simulink model "sequentialProcessorNarenKolli"  (R2018b)
settings: Solver=VariableStepAuto  StartTime=0.0  StopTime=10  RelTol=1e-3
libraries: hdlsllib x172, simulink_extras x9
(part 2 of 4)

== system sequentialProcessorNarenKolli/8-Bit_Processor /8-Bit_Subtractor/Full Adder 6  ==
  X : Inport
  Y : Inport  Port=2
  Z : Inport  Port=3
  Half Adder : Subsystem
  Half Adder1 : Subsystem
  OR : Logic  Operator=OR  AllPortsSameDT=off  OutDataTypeStr=boolean
  S : Outport
  C : Outport  Port=2
  wires:
  Half Adder/2(Carry) -> OR/2
  OR/1 -> C/1
  Z/1 -> Half Adder1/2(B)
  X/1 -> Half Adder/1(A)
  Half Adder1/1(Sum) -> S/1
  Half Adder/1(Sum) -> Half Adder1/1(A)
  Y/1 -> Half Adder/2(B)
  Half Adder1/2(Carry) -> OR/1

== system sequentialProcessorNarenKolli/8-Bit_Processor /8-Bit_Subtractor/Full Adder 7  ==
  X : Inport
  Y : Inport  Port=2
  Z : Inport  Port=3
  Half Adder : Subsystem
  Half Adder1 : Subsystem
  OR : Logic  Operator=OR  AllPortsSameDT=off  OutDataTypeStr=boolean
  S : Outport
  C : Outport  Port=2
  wires:
  Half Adder/2(Carry) -> OR/2
  OR/1 -> C/1
  Z/1 -> Half Adder1/2(B)
  X/1 -> Half Adder/1(A)
  Half Adder1/1(Sum) -> S/1
  Half Adder/1(Sum) -> Half Adder1/1(A)
  Y/1 -> Half Adder/2(B)
  Half Adder1/2(Carry) -> OR/1

== system sequentialProcessorNarenKolli/8-Bit_Processor /8-Bit_Subtractor/Slicer 1  ==
  X : Inport  OutDataTypeStr=uint8  SampleTime=1
  Bit Slice : hdlsllib/Logic and Bit Operations/Bit Slice  lidx=7  ridx=7
  Bit Slice1 : hdlsllib/Logic and Bit Operations/Bit Slice  lidx=6  ridx=6
  Bit Slice2 : hdlsllib/Logic and Bit Operations/Bit Slice  lidx=5  ridx=5
  Bit Slice3 : hdlsllib/Logic and Bit Operations/Bit Slice  lidx=4  ridx=4
  Bit Slice4 : hdlsllib/Logic and Bit Operations/Bit Slice  lidx=3  ridx=3
  Bit Slice5 : hdlsllib/Logic and Bit Operations/Bit Slice  lidx=2  ridx=2
  Bit Slice6 : hdlsllib/Logic and Bit Operations/Bit Slice  lidx=1  ridx=1
  Bit Slice7 : hdlsllib/Logic and Bit Operations/Bit Slice  lidx=0  ridx=0
  Data Type Conversion{,1..7} (8 alike) : DataTypeConversion
  Y7 : Outport
  Y6 : Outport  Port=2
  Y5 : Outport  Port=3
  Y4 : Outport  Port=4
  Y3 : Outport  Port=5
  Y2 : Outport  Port=6
  Y1 : Outport  Port=7
  Y0 : Outport  Port=8
  wires:
  Data Type Conversion4/1 -> Y4/1
  Bit Slice3/1 -> Data Type Conversion4/1
  X/1 -> Bit Slice3/1, Bit Slice2/1, Bit Slice1/1, Bit Slice/1, Bit Slice4/1, Bit Slice5/1, Bit Slice6/1, Bit Slice7/1
  Bit Slice1/1 -> Data Type Conversion6/1
  Data Type Conversion1/1 -> Y1/1
  Bit Slice6/1 -> Data Type Conversion1/1
  Bit Slice5/1 -> Data Type Conversion2/1
  Bit Slice2/1 -> Data Type Conversion5/1
  Data Type Conversion/1 -> Y0/1
  Bit Slice4/1 -> Data Type Conversion3/1
  Bit Slice/1 -> Data Type Conversion7/1
  Data Type Conversion7/1 -> Y7/1
  Bit Slice7/1 -> Data Type Conversion/1
  Data Type Conversion3/1 -> Y3/1
  Data Type Conversion5/1 -> Y5/1
  Data Type Conversion6/1 -> Y6/1
  Data Type Conversion2/1 -> Y2/1

== system sequentialProcessorNarenKolli/8-Bit_Processor /8-Bit_Subtractor/Slicer 2  ==
  X : Inport  OutDataTypeStr=uint8  SampleTime=1
  Bit Slice : hdlsllib/Logic and Bit Operations/Bit Slice  lidx=7  ridx=7
  Bit Slice1 : hdlsllib/Logic and Bit Operations/Bit Slice  lidx=6  ridx=6
  Bit Slice2 : hdlsllib/Logic and Bit Operations/Bit Slice  lidx=5  ridx=5
  Bit Slice3 : hdlsllib/Logic and Bit Operations/Bit Slice  lidx=4  ridx=4
  Bit Slice4 : hdlsllib/Logic and Bit Operations/Bit Slice  lidx=3  ridx=3
  Bit Slice5 : hdlsllib/Logic and Bit Operations/Bit Slice  lidx=2  ridx=2
  Bit Slice6 : hdlsllib/Logic and Bit Operations/Bit Slice  lidx=1  ridx=1
  Bit Slice7 : hdlsllib/Logic and Bit Operations/Bit Slice  lidx=0  ridx=0
  Data Type Conversion{,1..7} (8 alike) : DataTypeConversion
  Y7 : Outport
  Y6 : Outport  Port=2
  Y5 : Outport  Port=3
  Y4 : Outport  Port=4
  Y3 : Outport  Port=5
  Y2 : Outport  Port=6
  Y1 : Outport  Port=7
  Y0 : Outport  Port=8
  wires:
  Data Type Conversion4/1 -> Y4/1
  Bit Slice3/1 -> Data Type Conversion4/1
  X/1 -> Bit Slice3/1, Bit Slice2/1, Bit Slice1/1, Bit Slice/1, Bit Slice4/1, Bit Slice5/1, Bit Slice6/1, Bit Slice7/1
  Bit Slice1/1 -> Data Type Conversion6/1
  Data Type Conversion1/1 -> Y1/1
  Bit Slice6/1 -> Data Type Conversion1/1
  Bit Slice5/1 -> Data Type Conversion2/1
  Bit Slice2/1 -> Data Type Conversion5/1
  Data Type Conversion/1 -> Y0/1
  Bit Slice4/1 -> Data Type Conversion3/1
  Bit Slice/1 -> Data Type Conversion7/1
  Data Type Conversion7/1 -> Y7/1
  Bit Slice7/1 -> Data Type Conversion/1
  Data Type Conversion3/1 -> Y3/1
  Data Type Conversion5/1 -> Y5/1
  Data Type Conversion6/1 -> Y6/1
  Data Type Conversion2/1 -> Y2/1

== system sequentialProcessorNarenKolli/8-Bit_Processor /8-bit 4-to-1 MUX/4 x 1 MUX ==
  s : Inport  OutDataTypeStr=int8  SampleTime=1
  "x0 " : Inport  Port=2  OutDataTypeStr=boolean
  x2 : Inport  Port=3  OutDataTypeStr=boolean
  x1 : Inport  Port=4  OutDataTypeStr=boolean
  x3 : Inport  Port=5  OutDataTypeStr=boolean
  AND{,1..3} (4 alike) : Logic  Inputs=3  IconShape=distinctive  AllPortsSameDT=off  OutDataTypeStr=boolean
  Bit Slice : hdlsllib/Logic and Bit Operations/Bit Slice  lidx=1  ridx=1
      settings: SourceProductName=Simulink  SourceProductBaseCode=SL
  Bit Slice1 : hdlsllib/Logic and Bit Operations/Bit Slice  lidx=0  ridx=0
      settings: SourceProductName=Simulink  SourceProductBaseCode=SL
  Data Type Conversion : DataTypeConversion  OutDataTypeStr=boolean
  Data Type Conversion1 : DataTypeConversion  OutDataTypeStr=boolean
  NOT S0 : Logic  Operator=NOT  IconShape=distinctive  AllPortsSameDT=off  OutDataTypeStr=boolean
  NOT S1 : Logic  Operator=NOT  IconShape=distinctive  AllPortsSameDT=off  OutDataTypeStr=boolean
  OR : Logic  Operator=OR  Inputs=4  IconShape=distinctive  AllPortsSameDT=off  OutDataTypeStr=boolean
  y : Outport  VectorParamsAs1DForOutWhenUnconnected=on
  wires:
  Data Type Conversion/1 -> AND3/1, AND2/1, NOT S1/1
  Data Type Conversion1/1 -> AND3/2, AND1/2, NOT S0/1
  NOT S0/1 -> AND2/2, AND/2
  x1/1 -> AND1/3
  x2/1 -> AND2/3
  AND3/1 -> OR/4
  NOT S1/1 -> AND1/1, AND/1
  x3/1 -> AND3/3
  AND2/1 -> OR/3
  AND1/1 -> OR/2
  "x0 "/1 -> AND/3
  Bit Slice1/1 -> Data Type Conversion1/1
  s/1 -> Bit Slice/1, Bit Slice1/1
  Bit Slice/1 -> Data Type Conversion/1
  AND/1 -> OR/1
  OR/1 -> y/1

== system sequentialProcessorNarenKolli/8-Bit_Processor /8-bit 4-to-1 MUX/4 x 1 MUX1 ==
  s : Inport  OutDataTypeStr=int8  SampleTime=1
  "x0 " : Inport  Port=2  OutDataTypeStr=boolean
  x2 : Inport  Port=3  OutDataTypeStr=boolean
  x1 : Inport  Port=4  OutDataTypeStr=boolean
  x3 : Inport  Port=5  OutDataTypeStr=boolean
  AND{,1..3} (4 alike) : Logic  Inputs=3  IconShape=distinctive  AllPortsSameDT=off  OutDataTypeStr=boolean
  Bit Slice : hdlsllib/Logic and Bit Operations/Bit Slice  lidx=1  ridx=1
      settings: SourceProductName=Simulink  SourceProductBaseCode=SL
  Bit Slice1 : hdlsllib/Logic and Bit Operations/Bit Slice  lidx=0  ridx=0
      settings: SourceProductName=Simulink  SourceProductBaseCode=SL
  Data Type Conversion : DataTypeConversion  OutDataTypeStr=boolean
  Data Type Conversion1 : DataTypeConversion  OutDataTypeStr=boolean
  NOT S0 : Logic  Operator=NOT  IconShape=distinctive  AllPortsSameDT=off  OutDataTypeStr=boolean
  NOT S1 : Logic  Operator=NOT  IconShape=distinctive  AllPortsSameDT=off  OutDataTypeStr=boolean
  OR : Logic  Operator=OR  Inputs=4  IconShape=distinctive  AllPortsSameDT=off  OutDataTypeStr=boolean
  y : Outport  VectorParamsAs1DForOutWhenUnconnected=on
  wires:
  Data Type Conversion/1 -> AND3/1, AND2/1, NOT S1/1
  Data Type Conversion1/1 -> AND3/2, AND1/2, NOT S0/1
  NOT S0/1 -> AND2/2, AND/2
  x1/1 -> AND1/3
  x2/1 -> AND2/3
  AND3/1 -> OR/4
  NOT S1/1 -> AND1/1, AND/1
  x3/1 -> AND3/3
  AND2/1 -> OR/3
  AND1/1 -> OR/2
  "x0 "/1 -> AND/3
  Bit Slice1/1 -> Data Type Conversion1/1
  s/1 -> Bit Slice/1, Bit Slice1/1
  Bit Slice/1 -> Data Type Conversion/1
  AND/1 -> OR/1
  OR/1 -> y/1

== system sequentialProcessorNarenKolli/8-Bit_Processor /8-bit 4-to-1 MUX/4 x 1 MUX2 ==
  s : Inport  OutDataTypeStr=int8  SampleTime=1
  "x0 " : Inport  Port=2  OutDataTypeStr=boolean
  x2 : Inport  Port=3  OutDataTypeStr=boolean
  x1 : Inport  Port=4  OutDataTypeStr=boolean
  x3 : Inport  Port=5  OutDataTypeStr=boolean
  AND{,1..3} (4 alike) : Logic  Inputs=3  IconShape=distinctive  AllPortsSameDT=off  OutDataTypeStr=boolean
  Bit Slice : hdlsllib/Logic and Bit Operations/Bit Slice  lidx=1  ridx=1
      settings: SourceProductName=Simulink  SourceProductBaseCode=SL
  Bit Slice1 : hdlsllib/Logic and Bit Operations/Bit Slice  lidx=0  ridx=0
      settings: SourceProductName=Simulink  SourceProductBaseCode=SL
  Data Type Conversion : DataTypeConversion  OutDataTypeStr=boolean
  Data Type Conversion1 : DataTypeConversion  OutDataTypeStr=boolean
  NOT S0 : Logic  Operator=NOT  IconShape=distinctive  AllPortsSameDT=off  OutDataTypeStr=boolean
  NOT S1 : Logic  Operator=NOT  IconShape=distinctive  AllPortsSameDT=off  OutDataTypeStr=boolean
  OR : Logic  Operator=OR  Inputs=4  IconShape=distinctive  AllPortsSameDT=off  OutDataTypeStr=boolean
  y : Outport  VectorParamsAs1DForOutWhenUnconnected=on
  wires:
  Data Type Conversion/1 -> AND3/1, AND2/1, NOT S1/1
  Data Type Conversion1/1 -> AND3/2, AND1/2, NOT S0/1
  NOT S0/1 -> AND2/2, AND/2
  x1/1 -> AND1/3
  x2/1 -> AND2/3
  AND3/1 -> OR/4
  NOT S1/1 -> AND1/1, AND/1
  x3/1 -> AND3/3
  AND2/1 -> OR/3
  AND1/1 -> OR/2
  "x0 "/1 -> AND/3
  Bit Slice1/1 -> Data Type Conversion1/1
  s/1 -> Bit Slice/1, Bit Slice1/1
  Bit Slice/1 -> Data Type Conversion/1
  AND/1 -> OR/1
  OR/1 -> y/1

== system sequentialProcessorNarenKolli/8-Bit_Processor /8-bit 4-to-1 MUX/4 x 1 MUX3 ==
  s : Inport  OutDataTypeStr=int8  SampleTime=1
  "x0 " : Inport  Port=2  OutDataTypeStr=boolean
  x2 : Inport  Port=3  OutDataTypeStr=boolean
  x1 : Inport  Port=4  OutDataTypeStr=boolean
  x3 : Inport  Port=5  OutDataTypeStr=boolean
  AND{,1..3} (4 alike) : Logic  Inputs=3  IconShape=distinctive  AllPortsSameDT=off  OutDataTypeStr=boolean
  Bit Slice : hdlsllib/Logic and Bit Operations/Bit Slice  lidx=1  ridx=1
      settings: SourceProductName=Simulink  SourceProductBaseCode=SL
  Bit Slice1 : hdlsllib/Logic and Bit Operations/Bit Slice  lidx=0  ridx=0
      settings: SourceProductName=Simulink  SourceProductBaseCode=SL
  Data Type Conversion : DataTypeConversion  OutDataTypeStr=boolean
  Data Type Conversion1 : DataTypeConversion  OutDataTypeStr=boolean
  NOT S0 : Logic  Operator=NOT  IconShape=distinctive  AllPortsSameDT=off  OutDataTypeStr=boolean
  NOT S1 : Logic  Operator=NOT  IconShape=distinctive  AllPortsSameDT=off  OutDataTypeStr=boolean
  OR : Logic  Operator=OR  Inputs=4  IconShape=distinctive  AllPortsSameDT=off  OutDataTypeStr=boolean
  y : Outport  VectorParamsAs1DForOutWhenUnconnected=on
  wires:
  Data Type Conversion/1 -> AND3/1, AND2/1, NOT S1/1
  Data Type Conversion1/1 -> AND3/2, AND1/2, NOT S0/1
  NOT S0/1 -> AND2/2, AND/2
  x1/1 -> AND1/3
  x2/1 -> AND2/3
  AND3/1 -> OR/4
  NOT S1/1 -> AND1/1, AND/1
  x3/1 -> AND3/3
  AND2/1 -> OR/3
  AND1/1 -> OR/2
  "x0 "/1 -> AND/3
  Bit Slice1/1 -> Data Type Conversion1/1
  s/1 -> Bit Slice/1, Bit Slice1/1
  Bit Slice/1 -> Data Type Conversion/1
  AND/1 -> OR/1
  OR/1 -> y/1

== system sequentialProcessorNarenKolli/8-Bit_Processor /8-bit 4-to-1 MUX/4 x 1 MUX4 ==
  s : Inport  OutDataTypeStr=int8  SampleTime=1
  "x0 " : Inport  Port=2  OutDataTypeStr=boolean
  x2 : Inport  Port=3  OutDataTypeStr=boolean
  x1 : Inport  Port=4  OutDataTypeStr=boolean
  x3 : Inport  Port=5  OutDataTypeStr=boolean
  AND{,1..3} (4 alike) : Logic  Inputs=3  IconShape=distinctive  AllPortsSameDT=off  OutDataTypeStr=boolean
  Bit Slice : hdlsllib/Logic and Bit Operations/Bit Slice  lidx=1  ridx=1
      settings: SourceProductName=Simulink  SourceProductBaseCode=SL
  Bit Slice1 : hdlsllib/Logic and Bit Operations/Bit Slice  lidx=0  ridx=0
      settings: SourceProductName=Simulink  SourceProductBaseCode=SL
  Data Type Conversion : DataTypeConversion  OutDataTypeStr=boolean
  Data Type Conversion1 : DataTypeConversion  OutDataTypeStr=boolean
  NOT S0 : Logic  Operator=NOT  IconShape=distinctive  AllPortsSameDT=off  OutDataTypeStr=boolean
  NOT S1 : Logic  Operator=NOT  IconShape=distinctive  AllPortsSameDT=off  OutDataTypeStr=boolean
  OR : Logic  Operator=OR  Inputs=4  IconShape=distinctive  AllPortsSameDT=off  OutDataTypeStr=boolean
  y : Outport  VectorParamsAs1DForOutWhenUnconnected=on
  wires:
  Data Type Conversion/1 -> AND3/1, AND2/1, NOT S1/1
  Data Type Conversion1/1 -> AND3/2, AND1/2, NOT S0/1
  NOT S0/1 -> AND2/2, AND/2
  x1/1 -> AND1/3
  x2/1 -> AND2/3
  AND3/1 -> OR/4
  NOT S1/1 -> AND1/1, AND/1
  x3/1 -> AND3/3
  AND2/1 -> OR/3
  AND1/1 -> OR/2
  "x0 "/1 -> AND/3
  Bit Slice1/1 -> Data Type Conversion1/1
  s/1 -> Bit Slice/1, Bit Slice1/1
  Bit Slice/1 -> Data Type Conversion/1
  AND/1 -> OR/1
  OR/1 -> y/1

== system sequentialProcessorNarenKolli/8-Bit_Processor /8-bit 4-to-1 MUX/4 x 1 MUX5 ==
  s : Inport  OutDataTypeStr=int8  SampleTime=1
  "x0 " : Inport  Port=2  OutDataTypeStr=boolean
  x2 : Inport  Port=3  OutDataTypeStr=boolean
  x1 : Inport  Port=4  OutDataTypeStr=boolean
  x3 : Inport  Port=5  OutDataTypeStr=boolean
  AND{,1..3} (4 alike) : Logic  Inputs=3  IconShape=distinctive  AllPortsSameDT=off  OutDataTypeStr=boolean
  Bit Slice : hdlsllib/Logic and Bit Operations/Bit Slice  lidx=1  ridx=1
      settings: SourceProductName=Simulink  SourceProductBaseCode=SL
  Bit Slice1 : hdlsllib/Logic and Bit Operations/Bit Slice  lidx=0  ridx=0
      settings: SourceProductName=Simulink  SourceProductBaseCode=SL
  Data Type Conversion : DataTypeConversion  OutDataTypeStr=boolean
  Data Type Conversion1 : DataTypeConversion  OutDataTypeStr=boolean
  NOT S0 : Logic  Operator=NOT  IconShape=distinctive  AllPortsSameDT=off  OutDataTypeStr=boolean
  NOT S1 : Logic  Operator=NOT  IconShape=distinctive  AllPortsSameDT=off  OutDataTypeStr=boolean
  OR : Logic  Operator=OR  Inputs=4  IconShape=distinctive  AllPortsSameDT=off  OutDataTypeStr=boolean
  y : Outport  VectorParamsAs1DForOutWhenUnconnected=on
  wires:
  Data Type Conversion/1 -> AND3/1, AND2/1, NOT S1/1
  Data Type Conversion1/1 -> AND3/2, AND1/2, NOT S0/1
  NOT S0/1 -> AND2/2, AND/2
  x1/1 -> AND1/3
  x2/1 -> AND2/3
  AND3/1 -> OR/4
  NOT S1/1 -> AND1/1, AND/1
  x3/1 -> AND3/3
  AND2/1 -> OR/3
  AND1/1 -> OR/2
  "x0 "/1 -> AND/3
  Bit Slice1/1 -> Data Type Conversion1/1
  s/1 -> Bit Slice/1, Bit Slice1/1
  Bit Slice/1 -> Data Type Conversion/1
  AND/1 -> OR/1
  OR/1 -> y/1

== system sequentialProcessorNarenKolli/8-Bit_Processor /8-bit 4-to-1 MUX/4 x 1 MUX6 ==
  s : Inport  OutDataTypeStr=int8  SampleTime=1
  "x0 " : Inport  Port=2  OutDataTypeStr=boolean
  x2 : Inport  Port=3  OutDataTypeStr=boolean
  x1 : Inport  Port=4  OutDataTypeStr=boolean
  x3 : Inport  Port=5  OutDataTypeStr=boolean
  AND{,1..3} (4 alike) : Logic  Inputs=3  IconShape=distinctive  AllPortsSameDT=off  OutDataTypeStr=boolean
  Bit Slice : hdlsllib/Logic and Bit Operations/Bit Slice  lidx=1  ridx=1
      settings: SourceProductName=Simulink  SourceProductBaseCode=SL
  Bit Slice1 : hdlsllib/Logic and Bit Operations/Bit Slice  lidx=0  ridx=0
      settings: SourceProductName=Simulink  SourceProductBaseCode=SL
  Data Type Conversion : DataTypeConversion  OutDataTypeStr=boolean
  Data Type Conversion1 : DataTypeConversion  OutDataTypeStr=boolean
  NOT S0 : Logic  Operator=NOT  IconShape=distinctive  AllPortsSameDT=off  OutDataTypeStr=boolean
  NOT S1 : Logic  Operator=NOT  IconShape=distinctive  AllPortsSameDT=off  OutDataTypeStr=boolean
  OR : Logic  Operator=OR  Inputs=4  IconShape=distinctive  AllPortsSameDT=off  OutDataTypeStr=boolean
  y : Outport  VectorParamsAs1DForOutWhenUnconnected=on
  wires:
  Data Type Conversion/1 -> AND3/1, AND2/1, NOT S1/1
  Data Type Conversion1/1 -> AND3/2, AND1/2, NOT S0/1
  NOT S0/1 -> AND2/2, AND/2
  x1/1 -> AND1/3
  x2/1 -> AND2/3
  AND3/1 -> OR/4
  NOT S1/1 -> AND1/1, AND/1
  x3/1 -> AND3/3
  AND2/1 -> OR/3
  AND1/1 -> OR/2
  "x0 "/1 -> AND/3
  Bit Slice1/1 -> Data Type Conversion1/1
  s/1 -> Bit Slice/1, Bit Slice1/1
  Bit Slice/1 -> Data Type Conversion/1
  AND/1 -> OR/1
  OR/1 -> y/1

== system sequentialProcessorNarenKolli/8-Bit_Processor /8-bit 4-to-1 MUX/4 x 1 MUX7 ==
  s : Inport  OutDataTypeStr=int8  SampleTime=1
  "x0 " : Inport  Port=2  OutDataTypeStr=boolean
  x2 : Inport  Port=3  OutDataTypeStr=boolean
  x1 : Inport  Port=4  OutDataTypeStr=boolean
  x3 : Inport  Port=5  OutDataTypeStr=boolean
  AND{,1..3} (4 alike) : Logic  Inputs=3  IconShape=distinctive  AllPortsSameDT=off  OutDataTypeStr=boolean
  Bit Slice : hdlsllib/Logic and Bit Operations/Bit Slice  lidx=1  ridx=1
      settings: SourceProductName=Simulink  SourceProductBaseCode=SL
  Bit Slice1 : hdlsllib/Logic and Bit Operations/Bit Slice  lidx=0  ridx=0
      settings: SourceProductName=Simulink  SourceProductBaseCode=SL
  Data Type Conversion : DataTypeConversion  OutDataTypeStr=boolean
  Data Type Conversion1 : DataTypeConversion  OutDataTypeStr=boolean
  NOT S0 : Logic  Operator=NOT  IconShape=distinctive  AllPortsSameDT=off  OutDataTypeStr=boolean
  NOT S1 : Logic  Operator=NOT  IconShape=distinctive  AllPortsSameDT=off  OutDataTypeStr=boolean
  OR : Logic  Operator=OR  Inputs=4  IconShape=distinctive  AllPortsSameDT=off  OutDataTypeStr=boolean
  y : Outport  VectorParamsAs1DForOutWhenUnconnected=on
  wires:
  Data Type Conversion/1 -> AND3/1, AND2/1, NOT S1/1
  Data Type Conversion1/1 -> AND3/2, AND1/2, NOT S0/1
  NOT S0/1 -> AND2/2, AND/2
  x1/1 -> AND1/3
  x2/1 -> AND2/3
  AND3/1 -> OR/4
  NOT S1/1 -> AND1/1, AND/1
  x3/1 -> AND3/3
  AND2/1 -> OR/3
  AND1/1 -> OR/2
  "x0 "/1 -> AND/3
  Bit Slice1/1 -> Data Type Conversion1/1
  s/1 -> Bit Slice/1, Bit Slice1/1
  Bit Slice/1 -> Data Type Conversion/1
  AND/1 -> OR/1
  OR/1 -> y/1

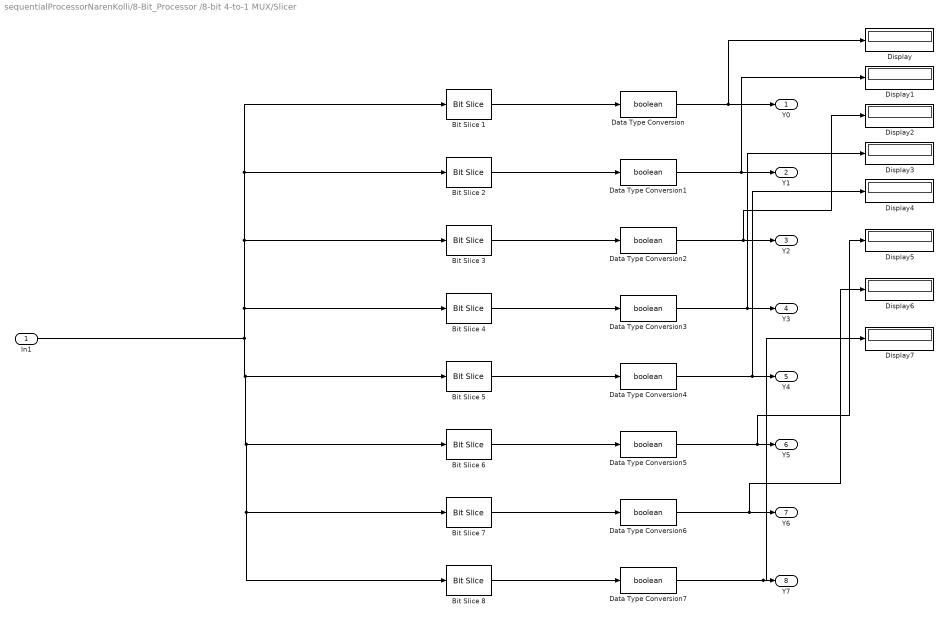
== system sequentialProcessorNarenKolli/8-Bit_Processor /8-bit 4-to-1 MUX/Slicer ==
  In1 : Inport
  Bit Slice 1 : hdlsllib/Logic and Bit Operations/Bit Slice  lidx=0  ridx=0
      settings: SourceProductName=Simulink  SourceProductBaseCode=SL
  "Bit Slice 2 " : hdlsllib/Logic and Bit Operations/Bit Slice  lidx=1  ridx=1
      settings: SourceProductName=Simulink  SourceProductBaseCode=SL
  Bit Slice 3 : hdlsllib/Logic and Bit Operations/Bit Slice  lidx=2  ridx=2
      settings: SourceProductName=Simulink  SourceProductBaseCode=SL
  Bit Slice 4 : hdlsllib/Logic and Bit Operations/Bit Slice  lidx=3  ridx=3
      settings: SourceProductName=Simulink  SourceProductBaseCode=SL
  Bit Slice 5 : hdlsllib/Logic and Bit Operations/Bit Slice  lidx=4  ridx=4
      settings: SourceProductName=Simulink  SourceProductBaseCode=SL
  Bit Slice 6 : hdlsllib/Logic and Bit Operations/Bit Slice  lidx=5  ridx=5
      settings: SourceProductName=Simulink  SourceProductBaseCode=SL
  Bit Slice 7 : hdlsllib/Logic and Bit Operations/Bit Slice  lidx=6  ridx=6
      settings: SourceProductName=Simulink  SourceProductBaseCode=SL
  Bit Slice 8 : hdlsllib/Logic and Bit Operations/Bit Slice  lidx=7  ridx=7
      settings: SourceProductName=Simulink  SourceProductBaseCode=SL
  Data Type Conversion{,1..7} (8 alike) : DataTypeConversion  OutDataTypeStr=boolean
  Display{,1..7} (8 alike) : Display
  Y0 : Outport  VectorParamsAs1DForOutWhenUnconnected=on
  Y1 : Outport  Port=2  VectorParamsAs1DForOutWhenUnconnected=on
  Y2 : Outport  Port=3  VectorParamsAs1DForOutWhenUnconnected=on
  Y3 : Outport  Port=4  VectorParamsAs1DForOutWhenUnconnected=on
  Y4 : Outport  Port=5  VectorParamsAs1DForOutWhenUnconnected=on
  Y5 : Outport  Port=6  VectorParamsAs1DForOutWhenUnconnected=on
  Y6 : Outport  Port=7  VectorParamsAs1DForOutWhenUnconnected=on
  Y7 : Outport  Port=8  VectorParamsAs1DForOutWhenUnconnected=on
  wires:
  Data Type Conversion2/1 -> Display2/1, Y2/1
  Data Type Conversion/1 -> Display/1, Y0/1
  Bit Slice 4/1 -> Data Type Conversion3/1
  Data Type Conversion7/1 -> Display7/1, Y7/1
  Bit Slice 3/1 -> Data Type Conversion2/1
  Bit Slice 8/1 -> Data Type Conversion7/1
  Bit Slice 1/1 -> Data Type Conversion/1
  Bit Slice 6/1 -> Data Type Conversion5/1
  Data Type Conversion1/1 -> Display1/1, Y1/1
  "Bit Slice 2 "/1 -> Data Type Conversion1/1
  Data Type Conversion3/1 -> Display3/1, Y3/1
  Data Type Conversion5/1 -> Display5/1, Y5/1
  Data Type Conversion6/1 -> Display6/1, Y6/1
  Data Type Conversion4/1 -> Display4/1, Y4/1
  Bit Slice 5/1 -> Data Type Conversion4/1
  Bit Slice 7/1 -> Data Type Conversion6/1
  In1/1 -> Bit Slice 4/1, Bit Slice 3/1, "Bit Slice 2 "/1, Bit Slice 1/1, Bit Slice 8/1, Bit Slice 7/1, Bit Slice 6/1, Bit Slice 5/1

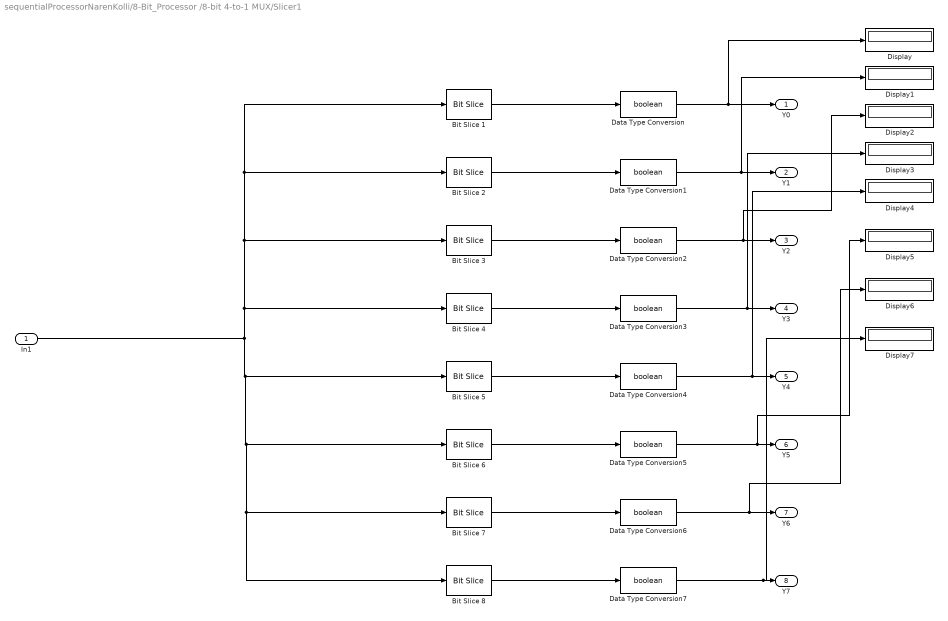
== system sequentialProcessorNarenKolli/8-Bit_Processor /8-bit 4-to-1 MUX/Slicer1 ==
  In1 : Inport
  Bit Slice 1 : hdlsllib/Logic and Bit Operations/Bit Slice  lidx=0  ridx=0
      settings: SourceProductName=Simulink  SourceProductBaseCode=SL
  "Bit Slice 2 " : hdlsllib/Logic and Bit Operations/Bit Slice  lidx=1  ridx=1
      settings: SourceProductName=Simulink  SourceProductBaseCode=SL
  Bit Slice 3 : hdlsllib/Logic and Bit Operations/Bit Slice  lidx=2  ridx=2
      settings: SourceProductName=Simulink  SourceProductBaseCode=SL
  Bit Slice 4 : hdlsllib/Logic and Bit Operations/Bit Slice  lidx=3  ridx=3
      settings: SourceProductName=Simulink  SourceProductBaseCode=SL
  Bit Slice 5 : hdlsllib/Logic and Bit Operations/Bit Slice  lidx=4  ridx=4
      settings: SourceProductName=Simulink  SourceProductBaseCode=SL
  Bit Slice 6 : hdlsllib/Logic and Bit Operations/Bit Slice  lidx=5  ridx=5
      settings: SourceProductName=Simulink  SourceProductBaseCode=SL
  Bit Slice 7 : hdlsllib/Logic and Bit Operations/Bit Slice  lidx=6  ridx=6
      settings: SourceProductName=Simulink  SourceProductBaseCode=SL
  Bit Slice 8 : hdlsllib/Logic and Bit Operations/Bit Slice  lidx=7  ridx=7
      settings: SourceProductName=Simulink  SourceProductBaseCode=SL
  Data Type Conversion{,1..7} (8 alike) : DataTypeConversion  OutDataTypeStr=boolean
  Display{,1..7} (8 alike) : Display
  Y0 : Outport  VectorParamsAs1DForOutWhenUnconnected=on
  Y1 : Outport  Port=2  VectorParamsAs1DForOutWhenUnconnected=on
  Y2 : Outport  Port=3  VectorParamsAs1DForOutWhenUnconnected=on
  Y3 : Outport  Port=4  VectorParamsAs1DForOutWhenUnconnected=on
  Y4 : Outport  Port=5  VectorParamsAs1DForOutWhenUnconnected=on
  Y5 : Outport  Port=6  VectorParamsAs1DForOutWhenUnconnected=on
  Y6 : Outport  Port=7  VectorParamsAs1DForOutWhenUnconnected=on
  Y7 : Outport  Port=8  VectorParamsAs1DForOutWhenUnconnected=on
  wires:
  Data Type Conversion2/1 -> Display2/1, Y2/1
  Data Type Conversion/1 -> Display/1, Y0/1
  Bit Slice 4/1 -> Data Type Conversion3/1
  Data Type Conversion7/1 -> Display7/1, Y7/1
  Bit Slice 3/1 -> Data Type Conversion2/1
  Bit Slice 8/1 -> Data Type Conversion7/1
  Bit Slice 1/1 -> Data Type Conversion/1
  Bit Slice 6/1 -> Data Type Conversion5/1
  Data Type Conversion1/1 -> Display1/1, Y1/1
  "Bit Slice 2 "/1 -> Data Type Conversion1/1
  Data Type Conversion3/1 -> Display3/1, Y3/1
  Data Type Conversion5/1 -> Display5/1, Y5/1
  Data Type Conversion6/1 -> Display6/1, Y6/1
  Data Type Conversion4/1 -> Display4/1, Y4/1
  Bit Slice 5/1 -> Data Type Conversion4/1
  Bit Slice 7/1 -> Data Type Conversion6/1
  In1/1 -> Bit Slice 4/1, Bit Slice 3/1, "Bit Slice 2 "/1, Bit Slice 1/1, Bit Slice 8/1, Bit Slice 7/1, Bit Slice 6/1, Bit Slice 5/1

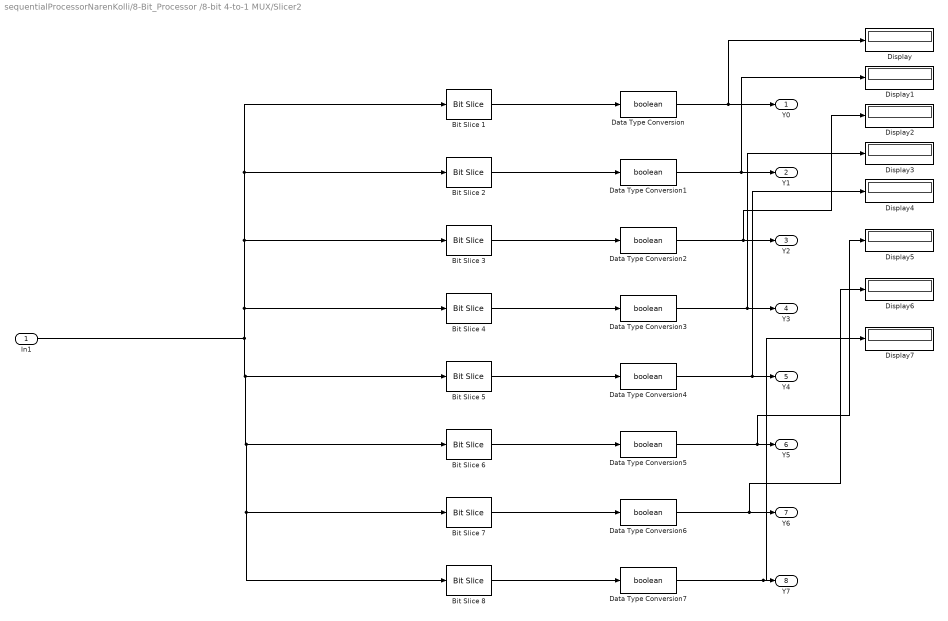
== system sequentialProcessorNarenKolli/8-Bit_Processor /8-bit 4-to-1 MUX/Slicer2 ==
  In1 : Inport
  Bit Slice 1 : hdlsllib/Logic and Bit Operations/Bit Slice  lidx=0  ridx=0
      settings: SourceProductName=Simulink  SourceProductBaseCode=SL
  "Bit Slice 2 " : hdlsllib/Logic and Bit Operations/Bit Slice  lidx=1  ridx=1
      settings: SourceProductName=Simulink  SourceProductBaseCode=SL
  Bit Slice 3 : hdlsllib/Logic and Bit Operations/Bit Slice  lidx=2  ridx=2
      settings: SourceProductName=Simulink  SourceProductBaseCode=SL
  Bit Slice 4 : hdlsllib/Logic and Bit Operations/Bit Slice  lidx=3  ridx=3
      settings: SourceProductName=Simulink  SourceProductBaseCode=SL
  Bit Slice 5 : hdlsllib/Logic and Bit Operations/Bit Slice  lidx=4  ridx=4
      settings: SourceProductName=Simulink  SourceProductBaseCode=SL
  Bit Slice 6 : hdlsllib/Logic and Bit Operations/Bit Slice  lidx=5  ridx=5
      settings: SourceProductName=Simulink  SourceProductBaseCode=SL
  Bit Slice 7 : hdlsllib/Logic and Bit Operations/Bit Slice  lidx=6  ridx=6
      settings: SourceProductName=Simulink  SourceProductBaseCode=SL
  Bit Slice 8 : hdlsllib/Logic and Bit Operations/Bit Slice  lidx=7  ridx=7
      settings: SourceProductName=Simulink  SourceProductBaseCode=SL
  Data Type Conversion{,1..7} (8 alike) : DataTypeConversion  OutDataTypeStr=boolean
  Display{,1..7} (8 alike) : Display
  Y0 : Outport  VectorParamsAs1DForOutWhenUnconnected=on
  Y1 : Outport  Port=2  VectorParamsAs1DForOutWhenUnconnected=on
  Y2 : Outport  Port=3  VectorParamsAs1DForOutWhenUnconnected=on
  Y3 : Outport  Port=4  VectorParamsAs1DForOutWhenUnconnected=on
  Y4 : Outport  Port=5  VectorParamsAs1DForOutWhenUnconnected=on
  Y5 : Outport  Port=6  VectorParamsAs1DForOutWhenUnconnected=on
  Y6 : Outport  Port=7  VectorParamsAs1DForOutWhenUnconnected=on
  Y7 : Outport  Port=8  VectorParamsAs1DForOutWhenUnconnected=on
  wires:
  Data Type Conversion2/1 -> Display2/1, Y2/1
  Data Type Conversion/1 -> Display/1, Y0/1
  Bit Slice 4/1 -> Data Type Conversion3/1
  Data Type Conversion7/1 -> Display7/1, Y7/1
  Bit Slice 3/1 -> Data Type Conversion2/1
  Bit Slice 8/1 -> Data Type Conversion7/1
  Bit Slice 1/1 -> Data Type Conversion/1
  Bit Slice 6/1 -> Data Type Conversion5/1
  Data Type Conversion1/1 -> Display1/1, Y1/1
  "Bit Slice 2 "/1 -> Data Type Conversion1/1
  Data Type Conversion3/1 -> Display3/1, Y3/1
  Data Type Conversion5/1 -> Display5/1, Y5/1
  Data Type Conversion6/1 -> Display6/1, Y6/1
  Data Type Conversion4/1 -> Display4/1, Y4/1
  Bit Slice 5/1 -> Data Type Conversion4/1
  Bit Slice 7/1 -> Data Type Conversion6/1
  In1/1 -> Bit Slice 4/1, Bit Slice 3/1, "Bit Slice 2 "/1, Bit Slice 1/1, Bit Slice 8/1, Bit Slice 7/1, Bit Slice 6/1, Bit Slice 5/1

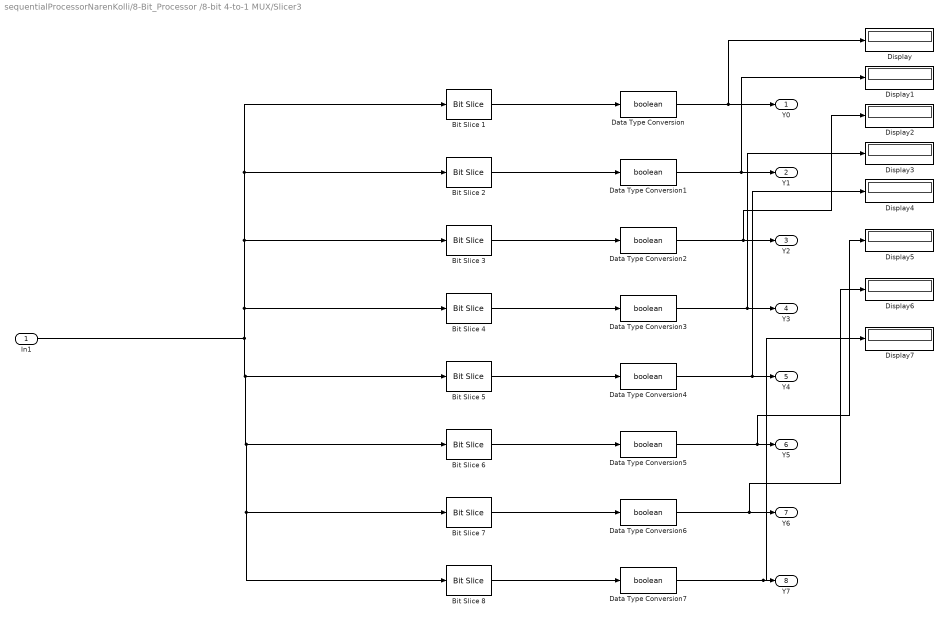
== system sequentialProcessorNarenKolli/8-Bit_Processor /8-bit 4-to-1 MUX/Slicer3 ==
  In1 : Inport
  Bit Slice 1 : hdlsllib/Logic and Bit Operations/Bit Slice  lidx=0  ridx=0
      settings: SourceProductName=Simulink  SourceProductBaseCode=SL
  "Bit Slice 2 " : hdlsllib/Logic and Bit Operations/Bit Slice  lidx=1  ridx=1
      settings: SourceProductName=Simulink  SourceProductBaseCode=SL
  Bit Slice 3 : hdlsllib/Logic and Bit Operations/Bit Slice  lidx=2  ridx=2
      settings: SourceProductName=Simulink  SourceProductBaseCode=SL
  Bit Slice 4 : hdlsllib/Logic and Bit Operations/Bit Slice  lidx=3  ridx=3
      settings: SourceProductName=Simulink  SourceProductBaseCode=SL
  Bit Slice 5 : hdlsllib/Logic and Bit Operations/Bit Slice  lidx=4  ridx=4
      settings: SourceProductName=Simulink  SourceProductBaseCode=SL
  Bit Slice 6 : hdlsllib/Logic and Bit Operations/Bit Slice  lidx=5  ridx=5
      settings: SourceProductName=Simulink  SourceProductBaseCode=SL
  Bit Slice 7 : hdlsllib/Logic and Bit Operations/Bit Slice  lidx=6  ridx=6
      settings: SourceProductName=Simulink  SourceProductBaseCode=SL
  Bit Slice 8 : hdlsllib/Logic and Bit Operations/Bit Slice  lidx=7  ridx=7
      settings: SourceProductName=Simulink  SourceProductBaseCode=SL
  Data Type Conversion{,1..7} (8 alike) : DataTypeConversion  OutDataTypeStr=boolean
  Display{,1..7} (8 alike) : Display
  Y0 : Outport  VectorParamsAs1DForOutWhenUnconnected=on
  Y1 : Outport  Port=2  VectorParamsAs1DForOutWhenUnconnected=on
  Y2 : Outport  Port=3  VectorParamsAs1DForOutWhenUnconnected=on
  Y3 : Outport  Port=4  VectorParamsAs1DForOutWhenUnconnected=on
  Y4 : Outport  Port=5  VectorParamsAs1DForOutWhenUnconnected=on
  Y5 : Outport  Port=6  VectorParamsAs1DForOutWhenUnconnected=on
  Y6 : Outport  Port=7  VectorParamsAs1DForOutWhenUnconnected=on
  Y7 : Outport  Port=8  VectorParamsAs1DForOutWhenUnconnected=on
  wires:
  Data Type Conversion2/1 -> Display2/1, Y2/1
  Data Type Conversion/1 -> Display/1, Y0/1
  Bit Slice 4/1 -> Data Type Conversion3/1
  Data Type Conversion7/1 -> Display7/1, Y7/1
  Bit Slice 3/1 -> Data Type Conversion2/1
  Bit Slice 8/1 -> Data Type Conversion7/1
  Bit Slice 1/1 -> Data Type Conversion/1
  Bit Slice 6/1 -> Data Type Conversion5/1
  Data Type Conversion1/1 -> Display1/1, Y1/1
  "Bit Slice 2 "/1 -> Data Type Conversion1/1
  Data Type Conversion3/1 -> Display3/1, Y3/1
  Data Type Conversion5/1 -> Display5/1, Y5/1
  Data Type Conversion6/1 -> Display6/1, Y6/1
  Data Type Conversion4/1 -> Display4/1, Y4/1
  Bit Slice 5/1 -> Data Type Conversion4/1
  Bit Slice 7/1 -> Data Type Conversion6/1
  In1/1 -> Bit Slice 4/1, Bit Slice 3/1, "Bit Slice 2 "/1, Bit Slice 1/1, Bit Slice 8/1, Bit Slice 7/1, Bit Slice 6/1, Bit Slice 5/1

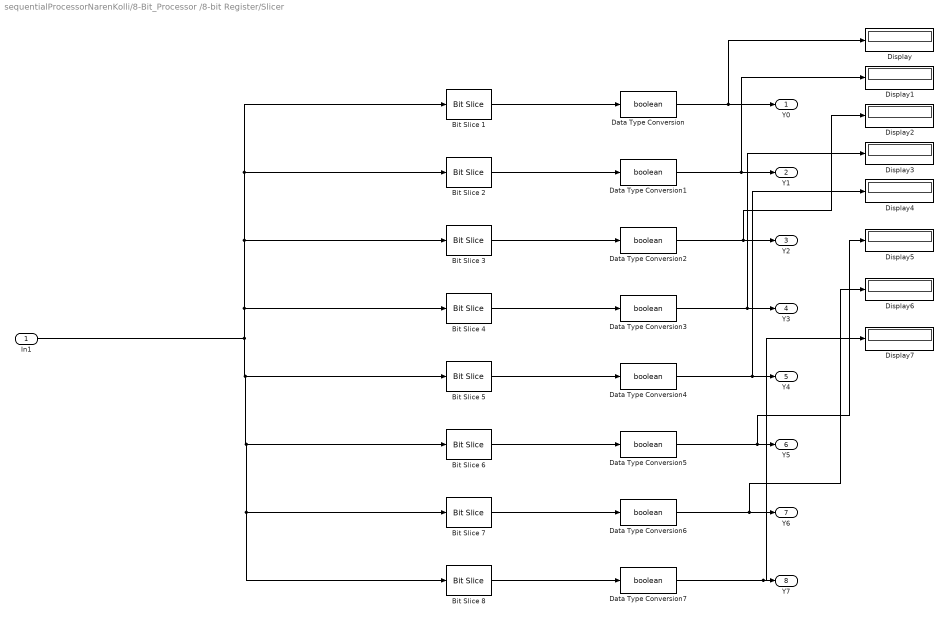
== system sequentialProcessorNarenKolli/8-Bit_Processor /8-bit Register/Slicer ==
  In1 : Inport
  Bit Slice 1 : hdlsllib/Logic and Bit Operations/Bit Slice  lidx=0  ridx=0
      settings: SourceProductName=Simulink  SourceProductBaseCode=SL
  "Bit Slice 2 " : hdlsllib/Logic and Bit Operations/Bit Slice  lidx=1  ridx=1
      settings: SourceProductName=Simulink  SourceProductBaseCode=SL
  Bit Slice 3 : hdlsllib/Logic and Bit Operations/Bit Slice  lidx=2  ridx=2
      settings: SourceProductName=Simulink  SourceProductBaseCode=SL
  Bit Slice 4 : hdlsllib/Logic and Bit Operations/Bit Slice  lidx=3  ridx=3
      settings: SourceProductName=Simulink  SourceProductBaseCode=SL
  Bit Slice 5 : hdlsllib/Logic and Bit Operations/Bit Slice  lidx=4  ridx=4
      settings: SourceProductName=Simulink  SourceProductBaseCode=SL
  Bit Slice 6 : hdlsllib/Logic and Bit Operations/Bit Slice  lidx=5  ridx=5
      settings: SourceProductName=Simulink  SourceProductBaseCode=SL
  Bit Slice 7 : hdlsllib/Logic and Bit Operations/Bit Slice  lidx=6  ridx=6
      settings: SourceProductName=Simulink  SourceProductBaseCode=SL
  Bit Slice 8 : hdlsllib/Logic and Bit Operations/Bit Slice  lidx=7  ridx=7
      settings: SourceProductName=Simulink  SourceProductBaseCode=SL
  Data Type Conversion{,1..7} (8 alike) : DataTypeConversion  OutDataTypeStr=boolean
  Display{,1..7} (8 alike) : Display
  Y0 : Outport  VectorParamsAs1DForOutWhenUnconnected=on
  Y1 : Outport  Port=2  VectorParamsAs1DForOutWhenUnconnected=on
  Y2 : Outport  Port=3  VectorParamsAs1DForOutWhenUnconnected=on
  Y3 : Outport  Port=4  VectorParamsAs1DForOutWhenUnconnected=on
  Y4 : Outport  Port=5  VectorParamsAs1DForOutWhenUnconnected=on
  Y5 : Outport  Port=6  VectorParamsAs1DForOutWhenUnconnected=on
  Y6 : Outport  Port=7  VectorParamsAs1DForOutWhenUnconnected=on
  Y7 : Outport  Port=8  VectorParamsAs1DForOutWhenUnconnected=on
  wires:
  Data Type Conversion2/1 -> Display2/1, Y2/1
  Data Type Conversion/1 -> Display/1, Y0/1
  Bit Slice 4/1 -> Data Type Conversion3/1
  Data Type Conversion7/1 -> Display7/1, Y7/1
  Bit Slice 3/1 -> Data Type Conversion2/1
  Bit Slice 8/1 -> Data Type Conversion7/1
  Bit Slice 1/1 -> Data Type Conversion/1
  Bit Slice 6/1 -> Data Type Conversion5/1
  Data Type Conversion1/1 -> Display1/1, Y1/1
  "Bit Slice 2 "/1 -> Data Type Conversion1/1
  Data Type Conversion3/1 -> Display3/1, Y3/1
  Data Type Conversion5/1 -> Display5/1, Y5/1
  Data Type Conversion6/1 -> Display6/1, Y6/1
  Data Type Conversion4/1 -> Display4/1, Y4/1
  Bit Slice 5/1 -> Data Type Conversion4/1
  Bit Slice 7/1 -> Data Type Conversion6/1
  In1/1 -> Bit Slice 4/1, Bit Slice 3/1, "Bit Slice 2 "/1, Bit Slice 1/1, Bit Slice 8/1, Bit Slice 7/1, Bit Slice 6/1, Bit Slice 5/1

== system sequentialProcessorNarenKolli/8-Bit_Processor /8-Bit_Adder/Full Adder 0 /Half Adder ==
  A : Inport
  B : Inport  Port=2
  AND (calculates carry) : Logic  AllPortsSameDT=off  OutDataTypeStr=boolean
  XOR (calculates sum) : Logic  Operator=XOR  AllPortsSameDT=off  OutDataTypeStr=boolean
  Sum : Outport
  Carry : Outport  Port=2
  wires:
  XOR (calculates sum)/1 -> Sum/1
  B/1 -> XOR (calculates sum)/2, AND (calculates carry)/2
  A/1 -> AND (calculates carry)/1, XOR (calculates sum)/1
  AND (calculates carry)/1 -> Carry/1

== system sequentialProcessorNarenKolli/8-Bit_Processor /8-Bit_Adder/Full Adder 0 /Half Adder1 ==
  A : Inport
  B : Inport  Port=2
  AND (calculates carry) : Logic  AllPortsSameDT=off  OutDataTypeStr=boolean
  XOR (calculates sum) : Logic  Operator=XOR  AllPortsSameDT=off  OutDataTypeStr=boolean
  Sum : Outport
  Carry : Outport  Port=2
  wires:
  XOR (calculates sum)/1 -> Sum/1
  B/1 -> XOR (calculates sum)/2, AND (calculates carry)/2
  A/1 -> AND (calculates carry)/1, XOR (calculates sum)/1
  AND (calculates carry)/1 -> Carry/1

== system sequentialProcessorNarenKolli/8-Bit_Processor /8-Bit_Adder/Full Adder 1 /Half Adder ==
  A : Inport
  B : Inport  Port=2
  AND (calculates carry) : Logic  AllPortsSameDT=off  OutDataTypeStr=boolean
  XOR (calculates sum) : Logic  Operator=XOR  AllPortsSameDT=off  OutDataTypeStr=boolean
  Sum : Outport
  Carry : Outport  Port=2
  wires:
  XOR (calculates sum)/1 -> Sum/1
  B/1 -> XOR (calculates sum)/2, AND (calculates carry)/2
  A/1 -> AND (calculates carry)/1, XOR (calculates sum)/1
  AND (calculates carry)/1 -> Carry/1

== system sequentialProcessorNarenKolli/8-Bit_Processor /8-Bit_Adder/Full Adder 1 /Half Adder1 ==
  A : Inport
  B : Inport  Port=2
  AND (calculates carry) : Logic  AllPortsSameDT=off  OutDataTypeStr=boolean
  XOR (calculates sum) : Logic  Operator=XOR  AllPortsSameDT=off  OutDataTypeStr=boolean
  Sum : Outport
  Carry : Outport  Port=2
  wires:
  XOR (calculates sum)/1 -> Sum/1
  B/1 -> XOR (calculates sum)/2, AND (calculates carry)/2
  A/1 -> AND (calculates carry)/1, XOR (calculates sum)/1
  AND (calculates carry)/1 -> Carry/1

== system sequentialProcessorNarenKolli/8-Bit_Processor /8-Bit_Adder/Full Adder 2 /Half Adder ==
  A : Inport
  B : Inport  Port=2
  AND (calculates carry) : Logic  AllPortsSameDT=off  OutDataTypeStr=boolean
  XOR (calculates sum) : Logic  Operator=XOR  AllPortsSameDT=off  OutDataTypeStr=boolean
  Sum : Outport
  Carry : Outport  Port=2
  wires:
  XOR (calculates sum)/1 -> Sum/1
  B/1 -> XOR (calculates sum)/2, AND (calculates carry)/2
  A/1 -> AND (calculates carry)/1, XOR (calculates sum)/1
  AND (calculates carry)/1 -> Carry/1

== system sequentialProcessorNarenKolli/8-Bit_Processor /8-Bit_Adder/Full Adder 2 /Half Adder1 ==
  A : Inport
  B : Inport  Port=2
  AND (calculates carry) : Logic  AllPortsSameDT=off  OutDataTypeStr=boolean
  XOR (calculates sum) : Logic  Operator=XOR  AllPortsSameDT=off  OutDataTypeStr=boolean
  Sum : Outport
  Carry : Outport  Port=2
  wires:
  XOR (calculates sum)/1 -> Sum/1
  B/1 -> XOR (calculates sum)/2, AND (calculates carry)/2
  A/1 -> AND (calculates carry)/1, XOR (calculates sum)/1
  AND (calculates carry)/1 -> Carry/1

== system sequentialProcessorNarenKolli/8-Bit_Processor /8-Bit_Adder/Full Adder 3 /Half Adder ==
  A : Inport
  B : Inport  Port=2
  AND (calculates carry) : Logic  AllPortsSameDT=off  OutDataTypeStr=boolean
  XOR (calculates sum) : Logic  Operator=XOR  AllPortsSameDT=off  OutDataTypeStr=boolean
  Sum : Outport
  Carry : Outport  Port=2
  wires:
  XOR (calculates sum)/1 -> Sum/1
  B/1 -> XOR (calculates sum)/2, AND (calculates carry)/2
  A/1 -> AND (calculates carry)/1, XOR (calculates sum)/1
  AND (calculates carry)/1 -> Carry/1

== system sequentialProcessorNarenKolli/8-Bit_Processor /8-Bit_Adder/Full Adder 3 /Half Adder1 ==
  A : Inport
  B : Inport  Port=2
  AND (calculates carry) : Logic  AllPortsSameDT=off  OutDataTypeStr=boolean
  XOR (calculates sum) : Logic  Operator=XOR  AllPortsSameDT=off  OutDataTypeStr=boolean
  Sum : Outport
  Carry : Outport  Port=2
  wires:
  XOR (calculates sum)/1 -> Sum/1
  B/1 -> XOR (calculates sum)/2, AND (calculates carry)/2
  A/1 -> AND (calculates carry)/1, XOR (calculates sum)/1
  AND (calculates carry)/1 -> Carry/1

== system sequentialProcessorNarenKolli/8-Bit_Processor /8-Bit_Adder/Full Adder 4 /Half Adder ==
  A : Inport
  B : Inport  Port=2
  AND (calculates carry) : Logic  AllPortsSameDT=off  OutDataTypeStr=boolean
  XOR (calculates sum) : Logic  Operator=XOR  AllPortsSameDT=off  OutDataTypeStr=boolean
  Sum : Outport
  Carry : Outport  Port=2
  wires:
  XOR (calculates sum)/1 -> Sum/1
  B/1 -> XOR (calculates sum)/2, AND (calculates carry)/2
  A/1 -> AND (calculates carry)/1, XOR (calculates sum)/1
  AND (calculates carry)/1 -> Carry/1

== system sequentialProcessorNarenKolli/8-Bit_Processor /8-Bit_Adder/Full Adder 4 /Half Adder1 ==
  A : Inport
  B : Inport  Port=2
  AND (calculates carry) : Logic  AllPortsSameDT=off  OutDataTypeStr=boolean
  XOR (calculates sum) : Logic  Operator=XOR  AllPortsSameDT=off  OutDataTypeStr=boolean
  Sum : Outport
  Carry : Outport  Port=2
  wires:
  XOR (calculates sum)/1 -> Sum/1
  B/1 -> XOR (calculates sum)/2, AND (calculates carry)/2
  A/1 -> AND (calculates carry)/1, XOR (calculates sum)/1
  AND (calculates carry)/1 -> Carry/1

== system sequentialProcessorNarenKolli/8-Bit_Processor /8-Bit_Adder/Full Adder 5 /Half Adder ==
  A : Inport
  B : Inport  Port=2
  AND (calculates carry) : Logic  AllPortsSameDT=off  OutDataTypeStr=boolean
  XOR (calculates sum) : Logic  Operator=XOR  AllPortsSameDT=off  OutDataTypeStr=boolean
  Sum : Outport
  Carry : Outport  Port=2
  wires:
  XOR (calculates sum)/1 -> Sum/1
  B/1 -> XOR (calculates sum)/2, AND (calculates carry)/2
  A/1 -> AND (calculates carry)/1, XOR (calculates sum)/1
  AND (calculates carry)/1 -> Carry/1

== system sequentialProcessorNarenKolli/8-Bit_Processor /8-Bit_Adder/Full Adder 5 /Half Adder1 ==
  A : Inport
  B : Inport  Port=2
  AND (calculates carry) : Logic  AllPortsSameDT=off  OutDataTypeStr=boolean
  XOR (calculates sum) : Logic  Operator=XOR  AllPortsSameDT=off  OutDataTypeStr=boolean
  Sum : Outport
  Carry : Outport  Port=2
  wires:
  XOR (calculates sum)/1 -> Sum/1
  B/1 -> XOR (calculates sum)/2, AND (calculates carry)/2
  A/1 -> AND (calculates carry)/1, XOR (calculates sum)/1
  AND (calculates carry)/1 -> Carry/1

== system sequentialProcessorNarenKolli/8-Bit_Processor /8-Bit_Adder/Full Adder 6 /Half Adder ==
  A : Inport
  B : Inport  Port=2
  AND (calculates carry) : Logic  AllPortsSameDT=off  OutDataTypeStr=boolean
  XOR (calculates sum) : Logic  Operator=XOR  AllPortsSameDT=off  OutDataTypeStr=boolean
  Sum : Outport
  Carry : Outport  Port=2
  wires:
  XOR (calculates sum)/1 -> Sum/1
  B/1 -> XOR (calculates sum)/2, AND (calculates carry)/2
  A/1 -> AND (calculates carry)/1, XOR (calculates sum)/1
  AND (calculates carry)/1 -> Carry/1

== system sequentialProcessorNarenKolli/8-Bit_Processor /8-Bit_Adder/Full Adder 6 /Half Adder1 ==
  A : Inport
  B : Inport  Port=2
  AND (calculates carry) : Logic  AllPortsSameDT=off  OutDataTypeStr=boolean
  XOR (calculates sum) : Logic  Operator=XOR  AllPortsSameDT=off  OutDataTypeStr=boolean
  Sum : Outport
  Carry : Outport  Port=2
  wires:
  XOR (calculates sum)/1 -> Sum/1
  B/1 -> XOR (calculates sum)/2, AND (calculates carry)/2
  A/1 -> AND (calculates carry)/1, XOR (calculates sum)/1
  AND (calculates carry)/1 -> Carry/1

== system sequentialProcessorNarenKolli/8-Bit_Processor /8-Bit_Adder/Full Adder 7 /Half Adder ==
  A : Inport
  B : Inport  Port=2
  AND (calculates carry) : Logic  AllPortsSameDT=off  OutDataTypeStr=boolean
  XOR (calculates sum) : Logic  Operator=XOR  AllPortsSameDT=off  OutDataTypeStr=boolean
  Sum : Outport
  Carry : Outport  Port=2
  wires:
  XOR (calculates sum)/1 -> Sum/1
  B/1 -> XOR (calculates sum)/2, AND (calculates carry)/2
  A/1 -> AND (calculates carry)/1, XOR (calculates sum)/1
  AND (calculates carry)/1 -> Carry/1

== system sequentialProcessorNarenKolli/8-Bit_Processor /8-Bit_Adder/Full Adder 7 /Half Adder1 ==
  A : Inport
  B : Inport  Port=2
  AND (calculates carry) : Logic  AllPortsSameDT=off  OutDataTypeStr=boolean
  XOR (calculates sum) : Logic  Operator=XOR  AllPortsSameDT=off  OutDataTypeStr=boolean
  Sum : Outport
  Carry : Outport  Port=2
  wires:
  XOR (calculates sum)/1 -> Sum/1
  B/1 -> XOR (calculates sum)/2, AND (calculates carry)/2
  A/1 -> AND (calculates carry)/1, XOR (calculates sum)/1
  AND (calculates carry)/1 -> Carry/1

== system sequentialProcessorNarenKolli/8-Bit_Processor /8-Bit_Multiplier/First 4x4 Multiplier /Full Adder ==
  X : Inport
  Y : Inport  Port=2
  Z : Inport  Port=3
  Half Adder : Subsystem
  Half Adder1 : Subsystem
  OR : Logic  Operator=OR  AllPortsSameDT=off  OutDataTypeStr=boolean
  S : Outport
  C : Outport  Port=2
  wires:
  Half Adder/2(Carry) -> OR/2
  OR/1 -> C/1
  Z/1 -> Half Adder1/2(B)
  X/1 -> Half Adder/1(A)
  Half Adder1/1(Sum) -> S/1
  Half Adder/1(Sum) -> Half Adder1/1(A)
  Y/1 -> Half Adder/2(B)
  Half Adder1/2(Carry) -> OR/1

== system sequentialProcessorNarenKolli/8-Bit_Processor /8-Bit_Multiplier/First 4x4 Multiplier /Full Adder1 ==
  X : Inport
  Y : Inport  Port=2
  Z : Inport  Port=3
  Half Adder : Subsystem
  Half Adder1 : Subsystem
  OR : Logic  Operator=OR  AllPortsSameDT=off  OutDataTypeStr=boolean
  S : Outport
  C : Outport  Port=2
  wires:
  Half Adder/2(Carry) -> OR/2
  OR/1 -> C/1
  Z/1 -> Half Adder1/2(B)
  X/1 -> Half Adder/1(A)
  Half Adder1/1(Sum) -> S/1
  Half Adder/1(Sum) -> Half Adder1/1(A)
  Y/1 -> Half Adder/2(B)
  Half Adder1/2(Carry) -> OR/1

== system sequentialProcessorNarenKolli/8-Bit_Processor /8-Bit_Multiplier/First 4x4 Multiplier /Full Adder2 ==
  X : Inport
  Y : Inport  Port=2
  Z : Inport  Port=3
  Half Adder : Subsystem
  Half Adder1 : Subsystem
  OR : Logic  Operator=OR  AllPortsSameDT=off  OutDataTypeStr=boolean
  S : Outport
  C : Outport  Port=2
  wires:
  Half Adder/2(Carry) -> OR/2
  OR/1 -> C/1
  Z/1 -> Half Adder1/2(B)
  X/1 -> Half Adder/1(A)
  Half Adder1/1(Sum) -> S/1
  Half Adder/1(Sum) -> Half Adder1/1(A)
  Y/1 -> Half Adder/2(B)
  Half Adder1/2(Carry) -> OR/1

== system sequentialProcessorNarenKolli/8-Bit_Processor /8-Bit_Multiplier/First 4x4 Multiplier /Full Adder3 ==
  X : Inport
  Y : Inport  Port=2
  Z : Inport  Port=3
  Half Adder : Subsystem
  Half Adder1 : Subsystem
  OR : Logic  Operator=OR  AllPortsSameDT=off  OutDataTypeStr=boolean
  S : Outport
  C : Outport  Port=2
  wires:
  Half Adder/2(Carry) -> OR/2
  OR/1 -> C/1
  Z/1 -> Half Adder1/2(B)
  X/1 -> Half Adder/1(A)
  Half Adder1/1(Sum) -> S/1
  Half Adder/1(Sum) -> Half Adder1/1(A)
  Y/1 -> Half Adder/2(B)
  Half Adder1/2(Carry) -> OR/1

== system sequentialProcessorNarenKolli/8-Bit_Processor /8-Bit_Multiplier/First 4x4 Multiplier /Full Adder4 ==
  X : Inport
  Y : Inport  Port=2
  Z : Inport  Port=3
  Half Adder : Subsystem
  Half Adder1 : Subsystem
  OR : Logic  Operator=OR  AllPortsSameDT=off  OutDataTypeStr=boolean
  S : Outport
  C : Outport  Port=2
  wires:
  Half Adder/2(Carry) -> OR/2
  OR/1 -> C/1
  Z/1 -> Half Adder1/2(B)
  X/1 -> Half Adder/1(A)
  Half Adder1/1(Sum) -> S/1
  Half Adder/1(Sum) -> Half Adder1/1(A)
  Y/1 -> Half Adder/2(B)
  Half Adder1/2(Carry) -> OR/1

== system sequentialProcessorNarenKolli/8-Bit_Processor /8-Bit_Multiplier/First 4x4 Multiplier /Full Adder5 ==
  X : Inport
  Y : Inport  Port=2
  Z : Inport  Port=3
  Half Adder : Subsystem
  Half Adder1 : Subsystem
  OR : Logic  Operator=OR  AllPortsSameDT=off  OutDataTypeStr=boolean
  S : Outport
  C : Outport  Port=2
  wires:
  Half Adder/2(Carry) -> OR/2
  OR/1 -> C/1
  Z/1 -> Half Adder1/2(B)
  X/1 -> Half Adder/1(A)
  Half Adder1/1(Sum) -> S/1
  Half Adder/1(Sum) -> Half Adder1/1(A)
  Y/1 -> Half Adder/2(B)
  Half Adder1/2(Carry) -> OR/1

== system sequentialProcessorNarenKolli/8-Bit_Processor /8-Bit_Multiplier/First 4x4 Multiplier /Full Adder6 ==
  X : Inport
  Y : Inport  Port=2
  Z : Inport  Port=3
  Half Adder : Subsystem
  Half Adder1 : Subsystem
  OR : Logic  Operator=OR  AllPortsSameDT=off  OutDataTypeStr=boolean
  S : Outport
  C : Outport  Port=2
  wires:
  Half Adder/2(Carry) -> OR/2
  OR/1 -> C/1
  Z/1 -> Half Adder1/2(B)
  X/1 -> Half Adder/1(A)
  Half Adder1/1(Sum) -> S/1
  Half Adder/1(Sum) -> Half Adder1/1(A)
  Y/1 -> Half Adder/2(B)
  Half Adder1/2(Carry) -> OR/1

== system sequentialProcessorNarenKolli/8-Bit_Processor /8-Bit_Multiplier/First 4x4 Multiplier /Full Adder7 ==
  X : Inport
  Y : Inport  Port=2
  Z : Inport  Port=3
  Half Adder : Subsystem
  Half Adder1 : Subsystem
  OR : Logic  Operator=OR  AllPortsSameDT=off  OutDataTypeStr=boolean
  S : Outport
  C : Outport  Port=2
  wires:
  Half Adder/2(Carry) -> OR/2
  OR/1 -> C/1
  Z/1 -> Half Adder1/2(B)
  X/1 -> Half Adder/1(A)
  Half Adder1/1(Sum) -> S/1
  Half Adder/1(Sum) -> Half Adder1/1(A)
  Y/1 -> Half Adder/2(B)
  Half Adder1/2(Carry) -> OR/1

== system sequentialProcessorNarenKolli/8-Bit_Processor /8-Bit_Multiplier/First 4x4 Multiplier /Half Adder ==
  A : Inport
  B : Inport  Port=2
  AND (calculates carry) : Logic  AllPortsSameDT=off  OutDataTypeStr=boolean
  XOR (calculates sum) : Logic  Operator=XOR  AllPortsSameDT=off  OutDataTypeStr=boolean
  Sum : Outport
  Carry : Outport  Port=2
  wires:
  XOR (calculates sum)/1 -> Sum/1
  B/1 -> XOR (calculates sum)/2, AND (calculates carry)/2
  A/1 -> AND (calculates carry)/1, XOR (calculates sum)/1
  AND (calculates carry)/1 -> Carry/1

== system sequentialProcessorNarenKolli/8-Bit_Processor /8-Bit_Multiplier/First 4x4 Multiplier /Half Adder1 ==
  A : Inport
  B : Inport  Port=2
  AND (calculates carry) : Logic  AllPortsSameDT=off  OutDataTypeStr=boolean
  XOR (calculates sum) : Logic  Operator=XOR  AllPortsSameDT=off  OutDataTypeStr=boolean
  Sum : Outport
  Carry : Outport  Port=2
  wires:
  XOR (calculates sum)/1 -> Sum/1
  B/1 -> XOR (calculates sum)/2, AND (calculates carry)/2
  A/1 -> AND (calculates carry)/1, XOR (calculates sum)/1
  AND (calculates carry)/1 -> Carry/1

== system sequentialProcessorNarenKolli/8-Bit_Processor /8-Bit_Multiplier/First 4x4 Multiplier /Half Adder2 ==
  A : Inport
  B : Inport  Port=2
  AND (calculates carry) : Logic  AllPortsSameDT=off  OutDataTypeStr=boolean
  XOR (calculates sum) : Logic  Operator=XOR  AllPortsSameDT=off  OutDataTypeStr=boolean
  Sum : Outport
  Carry : Outport  Port=2
  wires:
  XOR (calculates sum)/1 -> Sum/1
  B/1 -> XOR (calculates sum)/2, AND (calculates carry)/2
  A/1 -> AND (calculates carry)/1, XOR (calculates sum)/1
  AND (calculates carry)/1 -> Carry/1

== system sequentialProcessorNarenKolli/8-Bit_Processor /8-Bit_Multiplier/First 4x4 Multiplier /Half Adder3 ==
  A : Inport
  B : Inport  Port=2
  AND (calculates carry) : Logic  AllPortsSameDT=off  OutDataTypeStr=boolean
  XOR (calculates sum) : Logic  Operator=XOR  AllPortsSameDT=off  OutDataTypeStr=boolean
  Sum : Outport
  Carry : Outport  Port=2
  wires:
  XOR (calculates sum)/1 -> Sum/1
  B/1 -> XOR (calculates sum)/2, AND (calculates carry)/2
  A/1 -> AND (calculates carry)/1, XOR (calculates sum)/1
  AND (calculates carry)/1 -> Carry/1

== system sequentialProcessorNarenKolli/8-Bit_Processor /8-Bit_Multiplier/First 8-Bit_Adder/Full Adder ==
  X : Inport
  Y : Inport  Port=2
  Z : Inport  Port=3
  Half Adder : Subsystem
  Half Adder1 : Subsystem
  OR : Logic  Operator=OR  AllPortsSameDT=off  OutDataTypeStr=boolean
  S : Outport
  C : Outport  Port=2
  wires:
  Half Adder/2(Carry) -> OR/2
  OR/1 -> C/1
  Z/1 -> Half Adder1/2(B)
  X/1 -> Half Adder/1(A)
  Half Adder1/1(Sum) -> S/1
  Half Adder/1(Sum) -> Half Adder1/1(A)
  Y/1 -> Half Adder/2(B)
  Half Adder1/2(Carry) -> OR/1

== system sequentialProcessorNarenKolli/8-Bit_Processor /8-Bit_Multiplier/First 8-Bit_Adder/Full Adder1 ==
  X : Inport
  Y : Inport  Port=2
  Z : Inport  Port=3
  Half Adder : Subsystem
  Half Adder1 : Subsystem
  OR : Logic  Operator=OR  AllPortsSameDT=off  OutDataTypeStr=boolean
  S : Outport
  C : Outport  Port=2
  wires:
  Half Adder/2(Carry) -> OR/2
  OR/1 -> C/1
  Z/1 -> Half Adder1/2(B)
  X/1 -> Half Adder/1(A)
  Half Adder1/1(Sum) -> S/1
  Half Adder/1(Sum) -> Half Adder1/1(A)
  Y/1 -> Half Adder/2(B)
  Half Adder1/2(Carry) -> OR/1

== system sequentialProcessorNarenKolli/8-Bit_Processor /8-Bit_Multiplier/First 8-Bit_Adder/Full Adder2 ==
  X : Inport
  Y : Inport  Port=2
  Z : Inport  Port=3
  Half Adder : Subsystem
  Half Adder1 : Subsystem
  OR : Logic  Operator=OR  AllPortsSameDT=off  OutDataTypeStr=boolean
  S : Outport
  C : Outport  Port=2
  wires:
  Half Adder/2(Carry) -> OR/2
  OR/1 -> C/1
  Z/1 -> Half Adder1/2(B)
  X/1 -> Half Adder/1(A)
  Half Adder1/1(Sum) -> S/1
  Half Adder/1(Sum) -> Half Adder1/1(A)
  Y/1 -> Half Adder/2(B)
  Half Adder1/2(Carry) -> OR/1

== system sequentialProcessorNarenKolli/8-Bit_Processor /8-Bit_Multiplier/First 8-Bit_Adder/Full Adder3 ==
  X : Inport
  Y : Inport  Port=2
  Z : Inport  Port=3
  Half Adder : Subsystem
  Half Adder1 : Subsystem
  OR : Logic  Operator=OR  AllPortsSameDT=off  OutDataTypeStr=boolean
  S : Outport
  C : Outport  Port=2
  wires:
  Half Adder/2(Carry) -> OR/2
  OR/1 -> C/1
  Z/1 -> Half Adder1/2(B)
  X/1 -> Half Adder/1(A)
  Half Adder1/1(Sum) -> S/1
  Half Adder/1(Sum) -> Half Adder1/1(A)
  Y/1 -> Half Adder/2(B)
  Half Adder1/2(Carry) -> OR/1

== system sequentialProcessorNarenKolli/8-Bit_Processor /8-Bit_Multiplier/First 8-Bit_Adder/Full Adder4 ==
  X : Inport
  Y : Inport  Port=2
  Z : Inport  Port=3
  Half Adder : Subsystem
  Half Adder1 : Subsystem
  OR : Logic  Operator=OR  AllPortsSameDT=off  OutDataTypeStr=boolean
  S : Outport
  C : Outport  Port=2
  wires:
  Half Adder/2(Carry) -> OR/2
  OR/1 -> C/1
  Z/1 -> Half Adder1/2(B)
  X/1 -> Half Adder/1(A)
  Half Adder1/1(Sum) -> S/1
  Half Adder/1(Sum) -> Half Adder1/1(A)
  Y/1 -> Half Adder/2(B)
  Half Adder1/2(Carry) -> OR/1
